simulink model "Mission_Server_Swarm_3QDrone_Vicon"  (Simulink 10.1)
settings: Solver=ode2  StartTime=0.0  StopTime=inf  FixedStep=0.001  RelTol=1e-3  EnableMultiTasking=on
undefined symbols (not defined in the file): datetime, Host, localhost, m, qc_get_step_size, saved_data
libraries: quarc_library x38, simulink x9
(part 1 of 2)
settings Model: Creator=Admin  LastModifiedBy=glai  SimulationMode=external  ExtModeTrigDuration=10000
settings SolverCC: PositivePriorityOrder=on
settings DataIOCC: SaveFormat=Dataset
settings OptimizationCC: LifeSpan=auto
settings DebuggingCC: UnderspecifiedInitializationDetection=Simplified  MergeDetectMultiDrivingBlocksExec=error
settings HardwareCC: ProdBitPerPointer=64  ProdBitPerSizeT=64  ProdBitPerPtrDiffT=64  ProdLargestAtomicFloat=Float  ProdIntDivRoundTo=Zero  ProdEndianess=LittleEndian  ProdWordSize=64  ProdHWDeviceType=Intel->x86-64 (Windows64)
settings ModelReferenceCC: PropagateSignalLabelsOutOfModel=on
settings RTWCC: Description=QUARC Win64 Target Using Toolchain  SystemTargetFile=quarc_win64.tlc  TemplateMakefile=quarc_default_tmf  Toolchain=QUARC win64 | nmake (64-bit Windows)  BuildConfiguration=Faster Runs
settings STFCustomTargetCC: ConcurrentExecutionCompliant=on  UseToolchainInfoCompliant=on  SystemTargetFile=quarc_win64.tlc
settings GRTTargetCC: ParMdlRefBuildCompliant=off  CompOptLevelCompliant=off  MatFileLogging=off  CPPClassGenCompliant=off  ExtMode=on  ExtModeMexFile=quarc_comm  ExtModeMexArgs='-w -d %d -uri %u -URI_Host_V1 tcpip://localhost:18001 -URI_Host_V2 tcpip://localhost:18002 -URI_Host_V3 tcpip://localhost:18003'

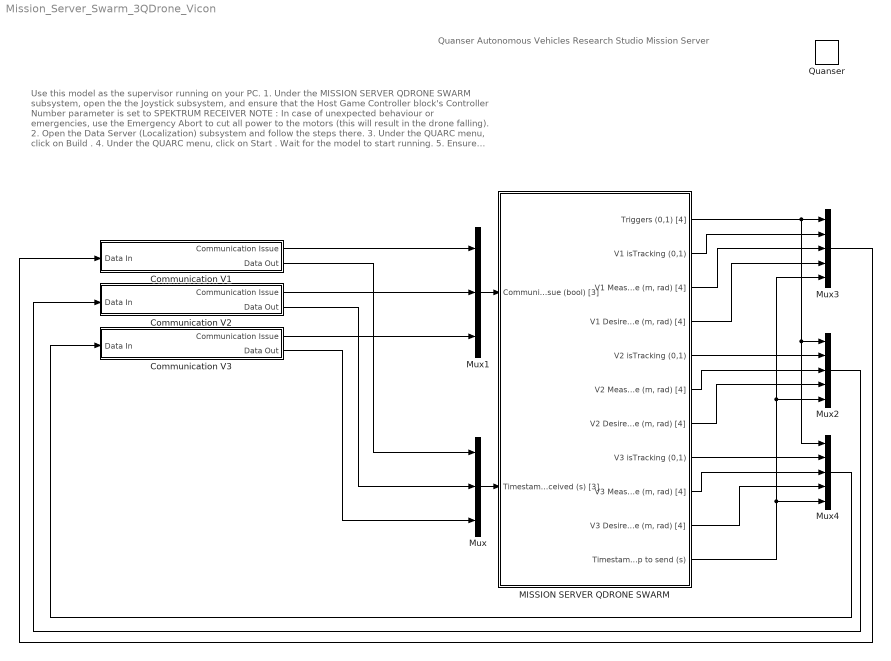
== system Mission_Server_Swarm_3QDrone_Vicon ==
  note: Use this model as the supervisor running on your PC.
      |
      | 1. Under the MISSION SERVER QDRONE SWARM subsystem, open the the Joystick subsystem, and ensure that the Host Game Controller block's Controller Number parameter is set to SPEKTRUM RECEIVER
      | NOTE : In case of unexpected behaviour or emergencies, use the Emergency Abort to cut all power to the motors (this will result in the drone falling).
      | 2. Open the Data Server (Localization) subsystem and follow the steps there.
      | 3. Under the QUARC menu, click on Build .
      | 4. Under the QUARC menu, click on Start . Wait for the model to start running.
      | 5. Ensure that the isTracking? display shows 1 and that the Joystick Issue display shows 0 (joystick must be powered ON with USB dongle attached to the PC).
      | NOTE : that the Comm Issue with Commander display SHOULD display 0 until the Commander_Stabilizer model is running. When it is running, this display should show 1.
  note: Quanser Autonomous Vehicles Research Studio
      | Mission Server
  Communication V1 : Subsystem
  Communication V2 : Subsystem
  Communication V3 : Subsystem
  MISSION SERVER QDRONE SWARM : Subsystem
  Mux : Mux  Inputs=3
  Mux1 : Mux  Inputs=3
  Mux2 : Mux  Inputs=5
  Mux3 : Mux  Inputs=5
  Mux4 : Mux  Inputs=5
  Quanser : quarc_library/Logos/Quanser
  wires:
  Communication V1/1(Communication Issue) -> Mux1/1
  Communication V2/1(Communication Issue) -> Mux1/2
  Communication V3/1(Communication Issue) -> Mux1/3
  Communication V3/2(Data Out) -> Mux/3
  Communication V2/2(Data Out) -> Mux/2
  Communication V1/2(Data Out) -> Mux/1
  MISSION SERVER QDRONE SWARM/11(Timestamp to send (s)) -> Mux3/5, Mux2/5, Mux4/5
  Mux3/1 -> Communication V1/1(Data In)
  Mux2/1 -> Communication V2/1(Data In)
  Mux4/1 -> Communication V3/1(Data In)
  Mux1/1 -> MISSION SERVER QDRONE SWARM/1(Communication  Issue (bool) [3])
  Mux/1 -> MISSION SERVER QDRONE SWARM/2(Timestamps received (s) [3])
  MISSION SERVER QDRONE SWARM/3("V1 Measured  Pose (m, rad) [4]") -> Mux3/3
  MISSION SERVER QDRONE SWARM/4("V1 Desired  Pose (m, rad) [4]") -> Mux3/4
  MISSION SERVER QDRONE SWARM/6("V2 Measured  Pose (m, rad) [4]") -> Mux2/3
  MISSION SERVER QDRONE SWARM/7("V2 Desired  Pose (m, rad) [4]") -> Mux2/4
  MISSION SERVER QDRONE SWARM/9("V3 Measured  Pose (m, rad) [4]") -> Mux4/3
  MISSION SERVER QDRONE SWARM/10("V3 Desired  Pose (m, rad) [4]") -> Mux4/4
  MISSION SERVER QDRONE SWARM/1(Triggers (0,1) [4]) -> Mux3/1, Mux4/1, Mux2/1
  MISSION SERVER QDRONE SWARM/2(V1 isTracking (0,1)) -> Mux3/2
  MISSION SERVER QDRONE SWARM/5(V2 isTracking (0,1)) -> Mux2/2
  MISSION SERVER QDRONE SWARM/8(V3 isTracking (0,1)) -> Mux4/2

== system Mission_Server_Swarm_3QDrone_Vicon/Communication V1 ==
  note: Argument (-URI_Host_V1) is set at the MEX-file arguments
      | found at Model Configuration Properties > Code Generation > Interface
      |
      | Format:
      | tcpip://localhost:18001
  Data In : Inport
  Constant : Constant
  Detect Communication loss : Subsystem
  Model Argument : quarc_library/Sources/Signals/Model Argument  argument_name=URI_Host_V1  has_value=on  data_type_mode=Specify via dialog  data_type=char  max_length=80  default_value=0  default_string=tcpip://localhost:18001  variable_size=off
      settings: AttributesFormatString=(-%<argument_name>)  SourceProductName=QUARC Targets
  Stream Server : quarc_library/Communications/Basic/Stream Server  uri_source=External input port  uri=tcpip://localhost:18877  apply_uri_to_all_configs=off  send_buffer_size=1460  receive_buffer_size=1460  byte_order=little endian (Intel - LSB first)  optimization=Minimum latency  send_options=Send most recent data  receive_options=Receive most recent data  default_value=zeros(1,1)  sample_time=qc_get_step_size  active=off  implementation=Use blocking I/O in a separate thread  send_fifo_size=1000  receive_fifo_size=1000  send_priority=0  receive_priority=0  send_dimensions=off  receive_dimensions=off  max_dimensions=-1  data_type=Inherited via back propagation  type_expr=BusObject
  "String Display " : quarc_library/Strings/String Display  alignment=center  display_mode=Single line  sample_time=-1  use_new=off
      settings: SourceProductName=QUARC Targets
  Terminator1 : Terminator
  Terminator2 : Terminator
  Communication Issue : Outport  VectorParamsAs1DForOutWhenUnconnected=off
  Data Out : Outport  Port=2  VectorParamsAs1DForOutWhenUnconnected=off
  wires:
  Detect Communication loss/1(Communication Issue (0,1)) -> Communication Issue/1
  Stream Server/1 -> Detect Communication loss/1(State)
  Stream Server/2 -> Detect Communication loss/2(Error)
  Stream Server/4 -> Data Out/1
  Model Argument/1 -> Stream Server/3, "String Display "/1
  Stream Server/5 -> Terminator1/1
  Stream Server/3 -> Terminator2/1
  Data In/1 -> Stream Server/1
  Constant/1 -> Stream Server/2

== system Mission_Server_Swarm_3QDrone_Vicon/Communication V2 ==
  note: Argument (-URI_Host_V2) is set at the MEX-file arguments
      | found at Model Configuration Properties > Code Generation > Interface
      |
      | Format:
      | tcpip://localhost:18002
  Data In : Inport
  Constant : Constant
  Detect Communication loss : Subsystem
  Model Argument : quarc_library/Sources/Signals/Model Argument  argument_name=URI_Host_V2  has_value=on  data_type_mode=Specify via dialog  data_type=char  max_length=80  default_value=0  default_string=tcpip://localhost:18002  variable_size=off
      settings: AttributesFormatString=(-%<argument_name>)  SourceProductName=QUARC Targets
  Stream Server : quarc_library/Communications/Basic/Stream Server  uri_source=External input port  uri=tcpip://localhost:18877  apply_uri_to_all_configs=off  send_buffer_size=1460  receive_buffer_size=1460  byte_order=little endian (Intel - LSB first)  optimization=Minimum latency  send_options=Send most recent data  receive_options=Receive most recent data  default_value=zeros(1,1)  sample_time=qc_get_step_size  active=off  implementation=Use blocking I/O in a separate thread  send_fifo_size=1000  receive_fifo_size=1000  send_priority=0  receive_priority=0  send_dimensions=off  receive_dimensions=off  max_dimensions=-1  data_type=Inherited via back propagation  type_expr=BusObject
  "String Display " : quarc_library/Strings/String Display  alignment=center  display_mode=Single line  sample_time=-1  use_new=off
      settings: SourceProductName=QUARC Targets
  Terminator1 : Terminator
  Terminator2 : Terminator
  Communication Issue : Outport  VectorParamsAs1DForOutWhenUnconnected=off
  Data Out : Outport  Port=2  VectorParamsAs1DForOutWhenUnconnected=off
  wires:
  Constant/1 -> Stream Server/2
  Data In/1 -> Stream Server/1
  Stream Server/3 -> Terminator2/1
  Stream Server/5 -> Terminator1/1
  Model Argument/1 -> "String Display "/1, Stream Server/3
  Stream Server/4 -> Data Out/1
  Stream Server/2 -> Detect Communication loss/2(Error)
  Stream Server/1 -> Detect Communication loss/1(State)
  Detect Communication loss/1(Communication Issue (0,1)) -> Communication Issue/1

== system Mission_Server_Swarm_3QDrone_Vicon/Communication V3 ==
  note: Argument (-URI_Host_V3) is set at the MEX-file arguments
      | found at Model Configuration Properties > Code Generation > Interface
      |
      | Format:
      | tcpip://localhost:18003
  Data In : Inport
  Constant : Constant
  Detect Communication loss : Subsystem
  Model Argument : quarc_library/Sources/Signals/Model Argument  argument_name=URI_Host_V3  has_value=on  data_type_mode=Specify via dialog  data_type=char  max_length=80  default_value=0  default_string=tcpip://localhost:18003  variable_size=off
      settings: AttributesFormatString=(-%<argument_name>)  SourceProductName=QUARC Targets
  Stream Server : quarc_library/Communications/Basic/Stream Server  uri_source=External input port  uri=tcpip://localhost:18877  apply_uri_to_all_configs=off  send_buffer_size=1460  receive_buffer_size=1460  byte_order=little endian (Intel - LSB first)  optimization=Minimum latency  send_options=Send most recent data  receive_options=Receive most recent data  default_value=zeros(1,1)  sample_time=qc_get_step_size  active=off  implementation=Use blocking I/O in a separate thread  send_fifo_size=1000  receive_fifo_size=1000  send_priority=0  receive_priority=0  send_dimensions=off  receive_dimensions=off  max_dimensions=-1  data_type=Inherited via back propagation  type_expr=BusObject
  "String Display " : quarc_library/Strings/String Display  alignment=center  display_mode=Single line  sample_time=-1  use_new=off
      settings: SourceProductName=QUARC Targets
  Terminator1 : Terminator
  Terminator2 : Terminator
  Communication Issue : Outport  VectorParamsAs1DForOutWhenUnconnected=off
  Data Out : Outport  Port=2  VectorParamsAs1DForOutWhenUnconnected=off
  wires:
  Detect Communication loss/1(Communication Issue (0,1)) -> Communication Issue/1
  Stream Server/1 -> Detect Communication loss/1(State)
  Stream Server/2 -> Detect Communication loss/2(Error)
  Stream Server/4 -> Data Out/1
  Model Argument/1 -> Stream Server/3, "String Display "/1
  Stream Server/5 -> Terminator1/1
  Stream Server/3 -> Terminator2/1
  Data In/1 -> Stream Server/1
  Constant/1 -> Stream Server/2

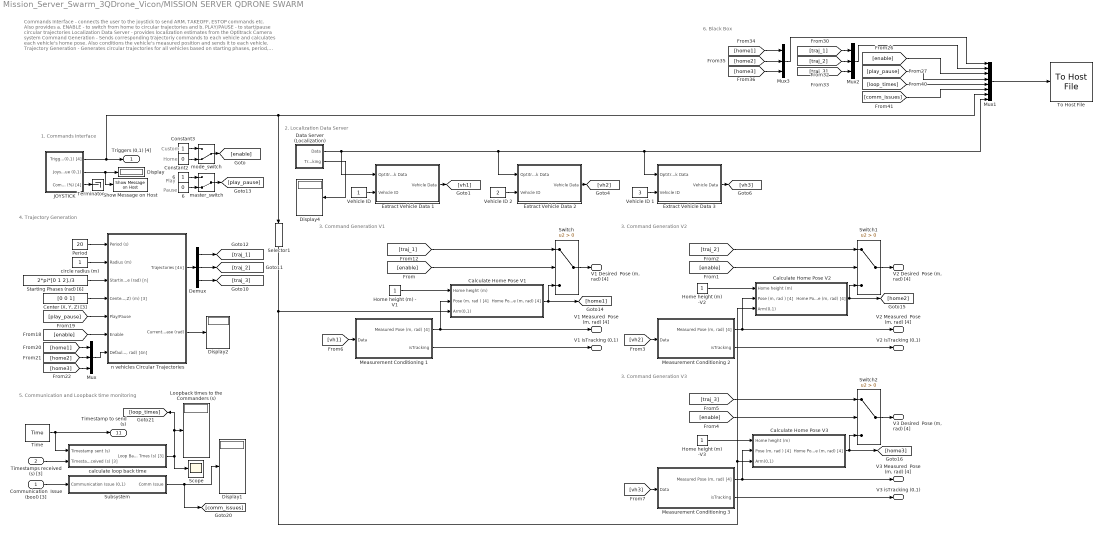
== system Mission_Server_Swarm_3QDrone_Vicon/MISSION SERVER QDRONE SWARM ==
  note: Commands Interface - connects the user to the joystick to send ARM, TAKEOFF, ESTOP commands etc. Also provides
      | a. ENABLE - to switch from home to circular trajectories and
      | b. PLAY/PAUSE - to start/pause circular trajectories
      | Localization Data Server - provides localization estimates from the Optitrack Camera system
      | Command Generation - Sends corresponding trajectoriy commands to each vehicle and calculates each vehicle's home pose. Also conditions the vehicle's measured position and sends it to each vehicle.
      | Trajectory Generation - Generates circular trajectories for all vehicles based on starting phases, period, radus and center location. When ENABLE is low, it switches to the trajectory at the Default (m, rad) [4] input
      | Communication and Loopback time monitoring - monitors communication issues with any vehicle, and also displays the loopback time to each model (time taken to send a packet to a vehicle and receive it back immediately).
      | Black Box: Logs selected data into log file for offline review and analysis.
  note: 6. Black Box
  note: 5. Communication and Loopback time monitoring
  note: 4. Trajectory Generation
  note: 2. Localization Data Server
  note: 1. Commands Interface
  note: Home
  note: Custom
  note: 3. Command Generation V1
  note: 3. Command Generation V2
  note: 3. Command Generation V3
  note: Pause
  note: Play
  Communication  Issue (bool) [3] : Inport
  Timestamps received (s) [3] : Inport  Port=2
  "          6" : Constant
  "   6" : Constant  Value=0
  Calculate Home Pose V1 : Subsystem
  Calculate Home Pose V2 : Subsystem
  Calculate Home Pose V3 : Subsystem
  "Center (X, Y, Z) [3]" : Constant  Value=[0 0 1]
  Constant2 : Constant  Value=0
  Constant3 : Constant
  "Data Server (Localization) " : Subsystem
  Demux : Demux  Outputs=[4 4 4 ]
  Display{,1..2,4} (4 alike) : Display
  Extract Vehicle Data 1 : Subsystem
  Extract Vehicle Data 2 : Subsystem
  Extract Vehicle Data 3 : Subsystem
  Home height (m) - V1 : Constant
  Home height (m) -V2 : Constant
  Home height (m) -V3 : Constant
  JOYSTICK : Subsystem
  Loopback times to the Commanders (s) : Display
  Measurement Conditioning 1 : Subsystem
  Measurement Conditioning 2 : Subsystem
  Measurement Conditioning 3 : Subsystem
  Mux : Mux  Inputs=3
  Mux1 : Mux  Inputs=8
  Mux2 : Mux  Inputs=3
  Mux3 : Mux  Inputs=3
  Period : Constant  Value=20
  Scope : Scope
  Selector1 : Selector  InputPortWidth=4  IndexOptions=Index vector (dialog)  Indices=[1]  OutputSizes=1
  "Show Message on Host " : quarc_library/Sinks/Error Handling/Show Message on Host  message_type=Fixed error message  message_icon=Warning  message=Mission Server: Joystick Disconnected
      settings: AttributesFormatString="\"%<message>\""  SourceProductName=QUARC Targets
  Starting Phases (rad) [6] : Constant  Value=2*pi*[0 1 2]./3
  Subsystem : Subsystem
  Switch : Switch  Criteria=u2 > Threshold
  Switch1 : Switch  Criteria=u2 > Threshold
  Switch2 : Switch  Criteria=u2 > Threshold
  Terminator : Terminator
  Time : quarc_library/Sources/Time/Time  time_source=Wall clock  sample_time=qc_get_step_size
  To Host File : quarc_library/Sinks/To Host/To Host File  file_name=saved_data/%m/%{char(datetime)}.mat  variable_name=data  decimation=1  sample_time=-1  file_format=MAT-file v.4  options=No header or footer  append=off  final_file_name=saved_data/Mission_Server_Swarm_3QDrone_Vicon/2022-03-11 10-34-30.mat  bitrate=2000000
  Vehicle ID : Constant
  Vehicle ID 1 : Constant  Value=3
  "Vehicle ID 2 " : Constant  Value=2
  calculate loop back time : Subsystem
  circle radius (m) : Constant
  master_switch : ManualSwitch  CurrentSetting=0
  mode_switch : ManualSwitch  CurrentSetting=0
  n vehicles Circular Trajectories : Subsystem
  Triggers (0,1) [4] : Outport  VectorParamsAs1DForOutWhenUnconnected=off
  V1 isTracking (0,1) : Outport  Port=2  VectorParamsAs1DForOutWhenUnconnected=off
  "V1 Measured  Pose (m, rad) [4]" : Outport  Port=3  VectorParamsAs1DForOutWhenUnconnected=off
  "V1 Desired  Pose (m, rad) [4]" : Outport  Port=4  VectorParamsAs1DForOutWhenUnconnected=off
  V2 isTracking (0,1) : Outport  Port=5  VectorParamsAs1DForOutWhenUnconnected=off
  "V2 Measured  Pose (m, rad) [4]" : Outport  Port=6  VectorParamsAs1DForOutWhenUnconnected=off
  "V2 Desired  Pose (m, rad) [4]" : Outport  Port=7  VectorParamsAs1DForOutWhenUnconnected=off
  V3 isTracking (0,1) : Outport  Port=8  VectorParamsAs1DForOutWhenUnconnected=off
  "V3 Measured  Pose (m, rad) [4]" : Outport  Port=9  VectorParamsAs1DForOutWhenUnconnected=off
  "V3 Desired  Pose (m, rad) [4]" : Outport  Port=10  VectorParamsAs1DForOutWhenUnconnected=off
  Timestamp to send (s) : Outport  Port=11  VectorParamsAs1DForOutWhenUnconnected=off
  wires:
  JOYSTICK/2(Joystick Issue (0,1)) -> Display/1, "Show Message on Host "/1
  Constant3/1 -> mode_switch/1
  Constant2/1 -> mode_switch/2
  JOYSTICK/3(Commands (%) [4]) -> Terminator/1
  "   6"/1 -> master_switch/2
  Period/1 -> n vehicles Circular Trajectories/1(Period (s))
  circle radius (m)/1 -> n vehicles Circular Trajectories/2(Radius (m))
  "          6"/1 -> master_switch/1
  [play_pause] -> n vehicles Circular Trajectories/5(Play/Pause)
  JOYSTICK/1(Triggers (0,1) [4]) -> Mux1/7, Selector1/1, Triggers (0,1) [4]/1
  "Data Server (Localization) "/2(Tracking) -> Display4/1
  Time/1 -> Timestamp to send (s)/1, calculate loop back time/1(Timestamp sent (s))
  Timestamps received (s) [3]/1 -> calculate loop back time/2(Timestamps received (s) [3])
  Starting Phases (rad) [6]/1 -> n vehicles Circular Trajectories/3(Starting Phase (rad) [n])
  "Center (X, Y, Z) [3]"/1 -> n vehicles Circular Trajectories/4(Center (X,Y,Z) (m) [3])
  n vehicles Circular Trajectories/2(Current Phase (rad)) -> Display2/1
  Vehicle ID 1/1 -> Extract Vehicle Data 3/2(Vehicle ID)
  "Vehicle ID 2 "/1 -> Extract Vehicle Data 2/2(Vehicle ID)
  Vehicle ID/1 -> Extract Vehicle Data 1/2(Vehicle ID)
  Measurement Conditioning 1/2(isTracking) -> V1 isTracking (0,1)/1
  Calculate Home Pose V1/1("Home Pose (m, rad) [4]") -> [home1], Switch/3
  [traj_1] -> Switch/1
  Home height (m) - V1/1 -> Calculate Home Pose V1/1(Home height (m))
  Measurement Conditioning 1/1("Measured Pose (m, rad) [4]") -> Calculate Home Pose V1/2("Pose (m, rad ) [4]"), "V1 Measured  Pose (m, rad) [4]"/1
  Switch/1 -> "V1 Desired  Pose (m, rad) [4]"/1
  mode_switch/1 -> [enable]
  [enable] -> Switch/2
  Extract Vehicle Data 1/1(Vehicle Data) -> [vh1]
  Extract Vehicle Data 2/1(Vehicle Data) -> [vh2]
  Extract Vehicle Data 3/1(Vehicle Data) -> [vh3]
  [vh1] -> Measurement Conditioning 1/1(Data)
  n vehicles Circular Trajectories/1(Trajectories [4n]) -> Demux/1
  Demux/1 -> [traj_1]
  Demux/2 -> [traj_2]
  Demux/3 -> [traj_3]
  [vh2] -> Measurement Conditioning 2/1(Data)
  [enable] -> Switch1/2
  Switch1/1 -> "V2 Desired  Pose (m, rad) [4]"/1
  Measurement Conditioning 2/1("Measured Pose (m, rad) [4]") -> Calculate Home Pose V2/2("Pose (m, rad ) [4]"), "V2 Measured  Pose (m, rad) [4]"/1
  Home height (m) -V2/1 -> Calculate Home Pose V2/1(Home height (m))
  [traj_2] -> Switch1/1
  Calculate Home Pose V2/1("Home Pose (m, rad) [4]") -> [home2], Switch1/3
  Measurement Conditioning 2/2(isTracking) -> V2 isTracking (0,1)/1
  Measurement Conditioning 3/2(isTracking) -> V3 isTracking (0,1)/1
  Calculate Home Pose V3/1("Home Pose (m, rad) [4]") -> [home3], Switch2/3
  [traj_3] -> Switch2/1
  Home height (m) -V3/1 -> Calculate Home Pose V3/1(Home height (m))
  Measurement Conditioning 3/1("Measured Pose (m, rad) [4]") -> Calculate Home Pose V3/2("Pose (m, rad ) [4]"), "V3 Measured  Pose (m, rad) [4]"/1
  Switch2/1 -> "V3 Desired  Pose (m, rad) [4]"/1
  [enable] -> Switch2/2
  [vh3] -> Measurement Conditioning 3/1(Data)
  [enable] -> n vehicles Circular Trajectories/6(Enable)
  master_switch/1 -> [play_pause]
  Communication  Issue (bool) [3]/1 -> Subsystem/1(Communication Issue (0,1))
  calculate loop back time/1(Loop Back Tmes (s) [3]) -> Scope/1, Loopback times to the Commanders (s)/1, [loop_times]
  Mux/1 -> n vehicles Circular Trajectories/7("Default (m, rad) [4n]")
  [home2] -> Mux/2
  [home3] -> Mux/3
  [home1] -> Mux/1
  Mux1/1 -> To Host File/1
  [play_pause] -> Mux1/4
  [enable] -> Mux1/3
  Mux2/1 -> Mux1/2
  [home1] -> Mux3/1
  [home3] -> Mux3/3
  [home2] -> Mux3/2
  [traj_3] -> Mux2/3
  [traj_2] -> Mux2/2
  [traj_1] -> Mux2/1
  Mux3/1 -> Mux1/1
  Subsystem/1(Comm Issue) -> [comm_issues], Display1/1
  [comm_issues] -> Mux1/6
  [loop_times] -> Mux1/5
  "Data Server (Localization) "/1(Data) -> Extract Vehicle Data 1/1(Optitrack Data), Extract Vehicle Data 2/1(Optitrack Data), Extract Vehicle Data 3/1(Optitrack Data), Mux1/8
  Selector1/1 -> Calculate Home Pose V3/3(Arm(0,1)), Calculate Home Pose V2/3(Arm(0,1)), Calculate Home Pose V1/3(Arm(0,1))

== system Mission_Server_Swarm_3QDrone_Vicon/Communication V1/Detect Communication loss ==
  State : Inport
  Error : Inport  Port=2
  Data Type Conversion : DataTypeConversion
  MATLAB Function : MATLAB Function  TreatAsAtomicUnit=on
  Terminator2 : Terminator
  Threshold : quarc_library/Discontinuities/Threshold  operator=>=  param_src=Specify via dialog  threshold=0.5  duration=0.1
      settings: SourceProductName=QUARC Targets
  Time : quarc_library/Sources/Time/Time  time_source=Wall clock  sample_time=qc_get_step_size
  Communication Issue (0,1) : Outport  VectorParamsAs1DForOutWhenUnconnected=off
  wires:
  Threshold/1 -> Data Type Conversion/1
  Data Type Conversion/1 -> Communication Issue (0,1)/1
  Threshold/2 -> Terminator2/1
  Time/1 -> MATLAB Function/1(time)
  State/1 -> MATLAB Function/2(state)
  MATLAB Function/1(stream_connection_loss) -> Threshold/1
  Error/1 -> MATLAB Function/3(error)

== system Mission_Server_Swarm_3QDrone_Vicon/Communication V2/Detect Communication loss ==
  State : Inport
  Error : Inport  Port=2
  Data Type Conversion : DataTypeConversion
  MATLAB Function : MATLAB Function  TreatAsAtomicUnit=on
  Terminator2 : Terminator
  Threshold : quarc_library/Discontinuities/Threshold  operator=>=  param_src=Specify via dialog  threshold=0.5  duration=0.1
      settings: SourceProductName=QUARC Targets
  Time : quarc_library/Sources/Time/Time  time_source=Wall clock  sample_time=qc_get_step_size
  Communication Issue (0,1) : Outport  VectorParamsAs1DForOutWhenUnconnected=off
  wires:
  Error/1 -> MATLAB Function/3(error)
  MATLAB Function/1(stream_connection_loss) -> Threshold/1
  State/1 -> MATLAB Function/2(state)
  Time/1 -> MATLAB Function/1(time)
  Threshold/2 -> Terminator2/1
  Data Type Conversion/1 -> Communication Issue (0,1)/1
  Threshold/1 -> Data Type Conversion/1

== system Mission_Server_Swarm_3QDrone_Vicon/Communication V3/Detect Communication loss ==
  State : Inport
  Error : Inport  Port=2
  Data Type Conversion : DataTypeConversion
  MATLAB Function : MATLAB Function  TreatAsAtomicUnit=on
  Terminator2 : Terminator
  Threshold : quarc_library/Discontinuities/Threshold  operator=>=  param_src=Specify via dialog  threshold=0.5  duration=0.1
      settings: SourceProductName=QUARC Targets
  Time : quarc_library/Sources/Time/Time  time_source=Wall clock  sample_time=qc_get_step_size
  Communication Issue (0,1) : Outport  VectorParamsAs1DForOutWhenUnconnected=off
  wires:
  Threshold/1 -> Data Type Conversion/1
  Data Type Conversion/1 -> Communication Issue (0,1)/1
  Threshold/2 -> Terminator2/1
  Time/1 -> MATLAB Function/1(time)
  State/1 -> MATLAB Function/2(state)
  MATLAB Function/1(stream_connection_loss) -> Threshold/1
  Error/1 -> MATLAB Function/3(error)

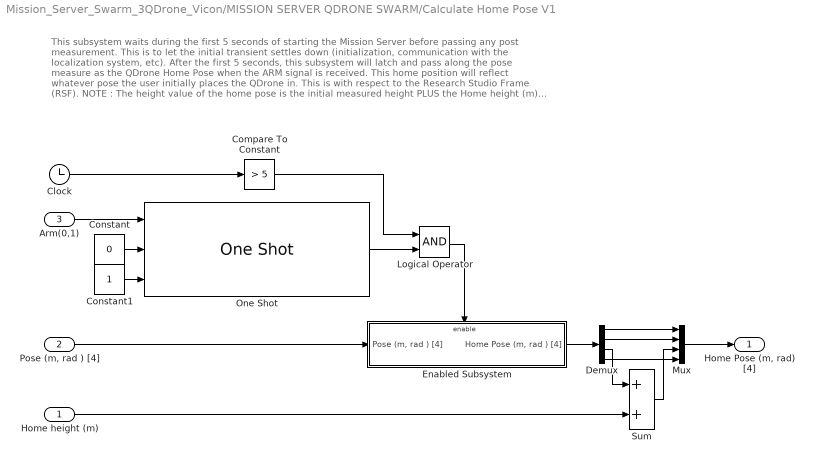
== system Mission_Server_Swarm_3QDrone_Vicon/MISSION SERVER QDRONE SWARM/Calculate Home Pose V1 ==
  note: This subsystem waits during the first 5 seconds of starting the Mission Server before passing any post measurement.
      | This is to let the initial transient settles down (initialization, communication with the localization system, etc).
      | After the first 5 seconds, this subsystem will latch and pass along the pose measure as the QDrone Home Pose when
      | the ARM signal is received.
      | This home position will reflect whatever pose the user initially places the QDrone in.
      | This is with respect to the Research Studio Frame (RSF).
      |
      | NOTE : The height value of the home pose is the initial measured height PLUS the Home height (m) input value.
  Home height (m) : Inport
  "Pose (m, rad ) [4]" : Inport  Port=2
  Arm(0,1) : Inport  Port=3
  Clock : Clock
  Compare To Constant : simulink/Logic and Bit Operations/Compare To Constant  relop=>  const=5  OutDataTypeStr=boolean
  Constant : Constant  Value=0
  Constant1 : Constant
  Demux : Demux
  Enabled Subsystem : Subsystem  TreatAsAtomicUnit=on
  Logical Operator : Logic  AllPortsSameDT=off  OutDataTypeStr=boolean
  Mux : Mux
  One Shot : quarc_library/Discontinuities/One Shot  trigger_type=Rising edge  redun_pulse=Ignore extraneous pulse  width_source=Specify via dialog  pulse_width=1/qc_get_step_size
      settings: SourceProductName=QUARC Targets
  Sum : Sum
  "Home Pose (m, rad) [4]" : Outport  VectorParamsAs1DForOutWhenUnconnected=off
  wires:
  Constant/1 -> One Shot/2
  Constant1/1 -> One Shot/3
  Arm(0,1)/1 -> One Shot/1
  One Shot/1 -> Logical Operator/2
  "Pose (m, rad ) [4]"/1 -> Enabled Subsystem/1("Pose (m, rad ) [4] ")
  Clock/1 -> Compare To Constant/1
  Compare To Constant/1 -> Logical Operator/1
  Logical Operator/1 -> Enabled Subsystem/Enable
  Enabled Subsystem/1("Home Pose (m, rad ) [4]") -> Demux/1
  Demux/1 -> Mux/1
  Demux/2 -> Mux/2
  Demux/4 -> Mux/4
  Demux/3 -> Sum/1
  Sum/1 -> Mux/3
  Home height (m)/1 -> Sum/2
  Mux/1 -> "Home Pose (m, rad) [4]"/1

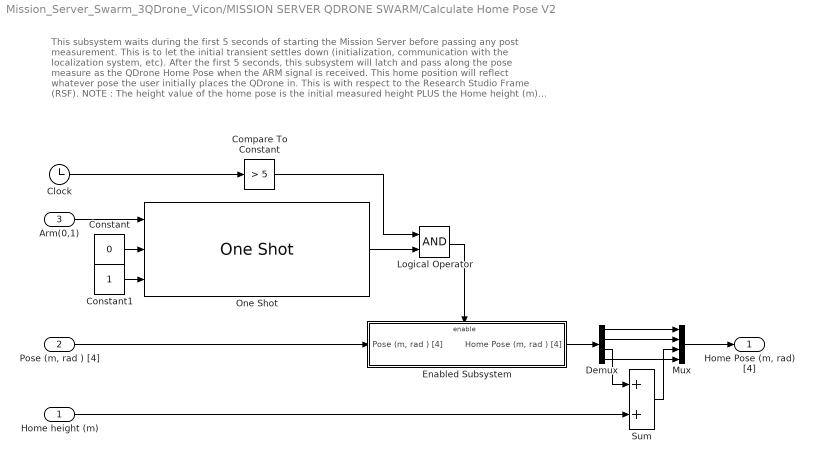
== system Mission_Server_Swarm_3QDrone_Vicon/MISSION SERVER QDRONE SWARM/Calculate Home Pose V2 ==
  note: This subsystem waits during the first 5 seconds of starting the Mission Server before passing any post measurement.
      | This is to let the initial transient settles down (initialization, communication with the localization system, etc).
      | After the first 5 seconds, this subsystem will latch and pass along the pose measure as the QDrone Home Pose when
      | the ARM signal is received.
      | This home position will reflect whatever pose the user initially places the QDrone in.
      | This is with respect to the Research Studio Frame (RSF).
      |
      | NOTE : The height value of the home pose is the initial measured height PLUS the Home height (m) input value.
  Home height (m) : Inport
  "Pose (m, rad ) [4]" : Inport  Port=2
  Arm(0,1) : Inport  Port=3
  Clock : Clock
  Compare To Constant : simulink/Logic and Bit Operations/Compare To Constant  relop=>  const=5  OutDataTypeStr=boolean
  Constant : Constant  Value=0
  Constant1 : Constant
  Demux : Demux
  Enabled Subsystem : Subsystem  TreatAsAtomicUnit=on
  Logical Operator : Logic  AllPortsSameDT=off  OutDataTypeStr=boolean
  Mux : Mux
  One Shot : quarc_library/Discontinuities/One Shot  trigger_type=Rising edge  redun_pulse=Ignore extraneous pulse  width_source=Specify via dialog  pulse_width=1/qc_get_step_size
      settings: SourceProductName=QUARC Targets
  Sum : Sum
  "Home Pose (m, rad) [4]" : Outport  VectorParamsAs1DForOutWhenUnconnected=off
  wires:
  Mux/1 -> "Home Pose (m, rad) [4]"/1
  Home height (m)/1 -> Sum/2
  Sum/1 -> Mux/3
  Demux/3 -> Sum/1
  Demux/4 -> Mux/4
  Demux/2 -> Mux/2
  Demux/1 -> Mux/1
  Enabled Subsystem/1("Home Pose (m, rad ) [4]") -> Demux/1
  Logical Operator/1 -> Enabled Subsystem/Enable
  Compare To Constant/1 -> Logical Operator/1
  Clock/1 -> Compare To Constant/1
  "Pose (m, rad ) [4]"/1 -> Enabled Subsystem/1("Pose (m, rad ) [4] ")
  One Shot/1 -> Logical Operator/2
  Arm(0,1)/1 -> One Shot/1
  Constant1/1 -> One Shot/3
  Constant/1 -> One Shot/2

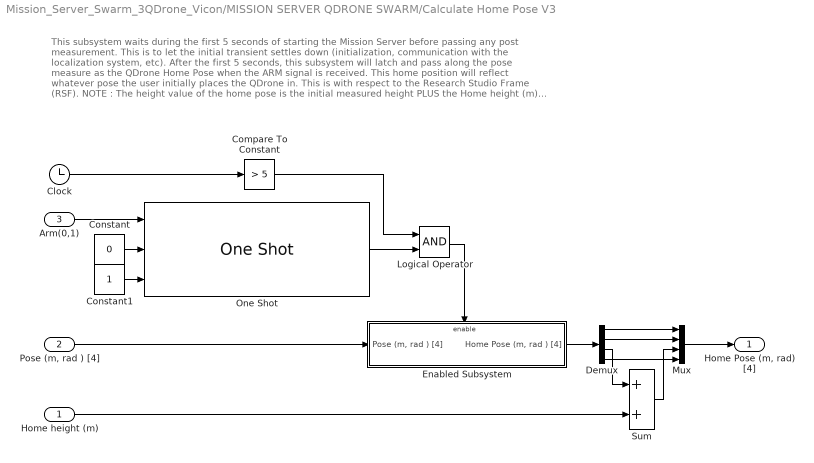
== system Mission_Server_Swarm_3QDrone_Vicon/MISSION SERVER QDRONE SWARM/Calculate Home Pose V3 ==
  note: This subsystem waits during the first 5 seconds of starting the Mission Server before passing any post measurement.
      | This is to let the initial transient settles down (initialization, communication with the localization system, etc).
      | After the first 5 seconds, this subsystem will latch and pass along the pose measure as the QDrone Home Pose when
      | the ARM signal is received.
      | This home position will reflect whatever pose the user initially places the QDrone in.
      | This is with respect to the Research Studio Frame (RSF).
      |
      | NOTE : The height value of the home pose is the initial measured height PLUS the Home height (m) input value.
  Home height (m) : Inport
  "Pose (m, rad ) [4]" : Inport  Port=2
  Arm(0,1) : Inport  Port=3
  Clock : Clock
  Compare To Constant : simulink/Logic and Bit Operations/Compare To Constant  relop=>  const=5  OutDataTypeStr=boolean
  Constant : Constant  Value=0
  Constant1 : Constant
  Demux : Demux
  Enabled Subsystem : Subsystem  TreatAsAtomicUnit=on
  Logical Operator : Logic  AllPortsSameDT=off  OutDataTypeStr=boolean
  Mux : Mux
  One Shot : quarc_library/Discontinuities/One Shot  trigger_type=Rising edge  redun_pulse=Ignore extraneous pulse  width_source=Specify via dialog  pulse_width=1/qc_get_step_size
      settings: SourceProductName=QUARC Targets
  Sum : Sum
  "Home Pose (m, rad) [4]" : Outport  VectorParamsAs1DForOutWhenUnconnected=off
  wires:
  Mux/1 -> "Home Pose (m, rad) [4]"/1
  Home height (m)/1 -> Sum/2
  Sum/1 -> Mux/3
  Demux/3 -> Sum/1
  Demux/4 -> Mux/4
  Demux/2 -> Mux/2
  Demux/1 -> Mux/1
  Enabled Subsystem/1("Home Pose (m, rad ) [4]") -> Demux/1
  Logical Operator/1 -> Enabled Subsystem/Enable
  Compare To Constant/1 -> Logical Operator/1
  Clock/1 -> Compare To Constant/1
  "Pose (m, rad ) [4]"/1 -> Enabled Subsystem/1("Pose (m, rad ) [4] ")
  One Shot/1 -> Logical Operator/2
  Arm(0,1)/1 -> One Shot/1
  Constant1/1 -> One Shot/3
  Constant/1 -> One Shot/2

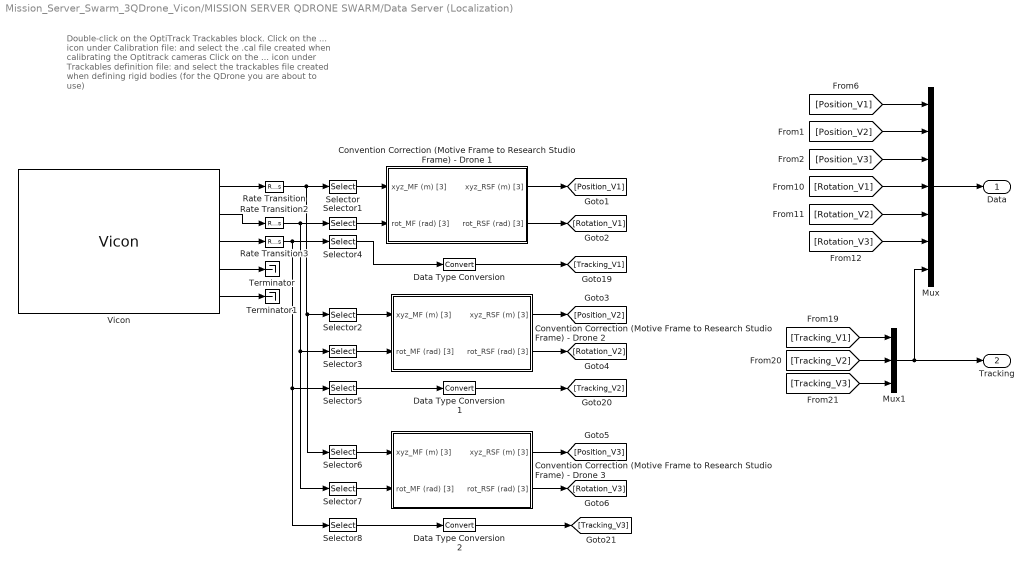
== system Mission_Server_Swarm_3QDrone_Vicon/MISSION SERVER QDRONE SWARM/Data Server (Localization)  ==
  note: Double-click on the OptiTrack Trackables block.
      |
      | Click on the ... icon under Calibration file: and select the .cal file
      | created when calibrating the Optitrack cameras
      |
      | Click on the ... icon under Trackables definition file: and select
      | the trackables file created when defining rigid bodies (for the
      | QDrone you are about to use)
  Convention Correction (Motive Frame to Research Studio Frame) - Drone 1 : Subsystem
  Convention Correction (Motive Frame to Research Studio Frame) - Drone 2 : Subsystem
  Convention Correction (Motive Frame to Research Studio Frame) - Drone 3 : Subsystem
  Data Type Conversion : DataTypeConversion
  Data Type Conversion1 : DataTypeConversion
  Data Type Conversion2 : DataTypeConversion
  Mux : Mux  Inputs=7
  Mux1 : Mux  Inputs=3
  Rate Transition : RateTransition
  Rate Transition2 : RateTransition
  Rate Transition3 : RateTransition
  Selector : Selector  InputPortWidth=9  IndexOptions=Index vector (dialog)  Indices=[1:3]  OutputSizes=1
  Selector1 : Selector  InputPortWidth=9  IndexOptions=Index vector (dialog)  Indices=[1:3]  OutputSizes=1
  Selector2 : Selector  InputPortWidth=9  IndexOptions=Index vector (dialog)  Indices=[4:6]  OutputSizes=1
  Selector3 : Selector  InputPortWidth=9  IndexOptions=Index vector (dialog)  Indices=[4:6]  OutputSizes=1
  Selector4 : Selector  InputPortWidth=3  IndexOptions=Index vector (dialog)  Indices=[1]  OutputSizes=1
  Selector5 : Selector  InputPortWidth=3  IndexOptions=Index vector (dialog)  Indices=[2]  OutputSizes=1
  Selector6 : Selector  InputPortWidth=9  IndexOptions=Index vector (dialog)  Indices=[7:9]  OutputSizes=1
  Selector7 : Selector  InputPortWidth=9  IndexOptions=Index vector (dialog)  Indices=[7:9]  OutputSizes=1
  Selector8 : Selector  InputPortWidth=3  IndexOptions=Index vector (dialog)  Indices=[3]  OutputSizes=1
  Terminator : Terminator
  Terminator1 : Terminator
  Vicon : quarc_library/Devices/Third-Party/Vicon/Vicon  hostname=localhost:801  segment_list=ObjectName.ObjectName\0ObjectName.ObjectName\0ObjectName.ObjectName\0\0  marker_list=\0  unlabeled_markers=[]  stream_mode=2  sample_time=qc_get_step_size  num_segments=3  num_markers=0  active=on
      settings: SourceProductName=QUARC Targets
  Data : Outport  VectorParamsAs1DForOutWhenUnconnected=off
  Tracking : Outport  Port=2  VectorParamsAs1DForOutWhenUnconnected=off
  wires:
  Vicon/3 -> Rate Transition3/1
  Mux/1 -> Data/1
  Vicon/1 -> Rate Transition/1
  Vicon/2 -> Rate Transition2/1
  Selector/1 -> Convention Correction (Motive Frame to Research Studio Frame) - Drone 1/1(xyz_MF (m) [3])
  Selector1/1 -> Convention Correction (Motive Frame to Research Studio Frame) - Drone 1/2(rot_MF (rad) [3])
  Selector2/1 -> Convention Correction (Motive Frame to Research Studio Frame) - Drone 2/1(xyz_MF (m) [3])
  Selector3/1 -> Convention Correction (Motive Frame to Research Studio Frame) - Drone 2/2(rot_MF (rad) [3])
  Selector4/1 -> Data Type Conversion/1
  Selector5/1 -> Data Type Conversion1/1
  Selector8/1 -> Data Type Conversion2/1
  Selector7/1 -> Convention Correction (Motive Frame to Research Studio Frame) - Drone 3/2(rot_MF (rad) [3])
  Selector6/1 -> Convention Correction (Motive Frame to Research Studio Frame) - Drone 3/1(xyz_MF (m) [3])
  Rate Transition2/1 -> Selector1/1, Selector7/1, Selector3/1
  Rate Transition3/1 -> Selector4/1, Selector8/1, Selector5/1
  Rate Transition/1 -> Selector6/1, Selector2/1, Selector/1
  Convention Correction (Motive Frame to Research Studio Frame) - Drone 1/1(xyz_RSF (m) [3]) -> [Position_V1]
  [Position_V1] -> Mux/1
  [Position_V2] -> Mux/2
  [Position_V3] -> Mux/3
  Convention Correction (Motive Frame to Research Studio Frame) - Drone 1/2(rot_RSF (rad) [3]) -> [Rotation_V1]
  [Rotation_V3] -> Mux/6
  [Tracking_V1] -> Mux1/1
  [Tracking_V2] -> Mux1/2
  [Tracking_V3] -> Mux1/3
  Convention Correction (Motive Frame to Research Studio Frame) - Drone 2/1(xyz_RSF (m) [3]) -> [Position_V2]
  Convention Correction (Motive Frame to Research Studio Frame) - Drone 2/2(rot_RSF (rad) [3]) -> [Rotation_V2]
  Convention Correction (Motive Frame to Research Studio Frame) - Drone 3/1(xyz_RSF (m) [3]) -> [Position_V3]
  Convention Correction (Motive Frame to Research Studio Frame) - Drone 3/2(rot_RSF (rad) [3]) -> [Rotation_V3]
  Data Type Conversion/1 -> [Tracking_V1]
  Data Type Conversion1/1 -> [Tracking_V2]
  Data Type Conversion2/1 -> [Tracking_V3]
  Mux1/1 -> Tracking/1, Mux/7
  [Rotation_V1] -> Mux/4
  [Rotation_V2] -> Mux/5
  Vicon/4 -> Terminator/1
  Vicon/5 -> Terminator1/1

== system Mission_Server_Swarm_3QDrone_Vicon/MISSION SERVER QDRONE SWARM/Extract Vehicle Data 1 ==
  Optitrack Data : Inport
  Vehicle ID : Inport  Port=2
  Data Type Conversion10 : DataTypeConversion
  Data Type Conversion11 : DataTypeConversion
  Data Type Conversion9 : DataTypeConversion
  Extract Object Data : MATLAB Function  TreatAsAtomicUnit=on
  Mux1 : Mux  Inputs=3
  Reshape : Reshape
  Reshape1 : Reshape
  Reshape2 : Reshape
  Vehicle Data : Outport  VectorParamsAs1DForOutWhenUnconnected=off
  wires:
  Reshape2/1 -> Data Type Conversion9/1
  Reshape1/1 -> Data Type Conversion10/1
  Reshape/1 -> Data Type Conversion11/1
  Data Type Conversion9/1 -> Mux1/3
  Data Type Conversion10/1 -> Mux1/2
  Data Type Conversion11/1 -> Mux1/1
  Extract Object Data/2(orientation) -> Reshape1/1
  Extract Object Data/3(tracking) -> Reshape2/1
  Extract Object Data/1(position) -> Reshape/1
  Mux1/1 -> Vehicle Data/1
  Optitrack Data/1 -> Extract Object Data/1(data)
  Vehicle ID/1 -> Extract Object Data/2(index)

== system Mission_Server_Swarm_3QDrone_Vicon/MISSION SERVER QDRONE SWARM/Extract Vehicle Data 2 ==
  Optitrack Data : Inport
  Vehicle ID : Inport  Port=2
  Data Type Conversion10 : DataTypeConversion
  Data Type Conversion11 : DataTypeConversion
  Data Type Conversion9 : DataTypeConversion
  Display : Display
  Display1 : Display
  Extract Object Data : MATLAB Function  TreatAsAtomicUnit=on
  Mux1 : Mux  Inputs=3
  Reshape : Reshape
  Reshape1 : Reshape
  Reshape2 : Reshape
  Vehicle Data : Outport  VectorParamsAs1DForOutWhenUnconnected=off
  wires:
  Vehicle ID/1 -> Extract Object Data/2(index)
  Optitrack Data/1 -> Extract Object Data/1(data)
  Mux1/1 -> Vehicle Data/1
  Extract Object Data/1(position) -> Display/1, Reshape/1
  Extract Object Data/3(tracking) -> Reshape2/1
  Extract Object Data/2(orientation) -> Display1/1, Reshape1/1
  Data Type Conversion11/1 -> Mux1/1
  Data Type Conversion10/1 -> Mux1/2
  Data Type Conversion9/1 -> Mux1/3
  Reshape/1 -> Data Type Conversion11/1
  Reshape1/1 -> Data Type Conversion10/1
  Reshape2/1 -> Data Type Conversion9/1

== system Mission_Server_Swarm_3QDrone_Vicon/MISSION SERVER QDRONE SWARM/Extract Vehicle Data 3 ==
  Optitrack Data : Inport
  Vehicle ID : Inport  Port=2
  Data Type Conversion10 : DataTypeConversion
  Data Type Conversion11 : DataTypeConversion
  Data Type Conversion9 : DataTypeConversion
  Extract Object Data : MATLAB Function  TreatAsAtomicUnit=on
  Mux1 : Mux  Inputs=3
  Reshape : Reshape
  Reshape1 : Reshape
  Reshape2 : Reshape
  Vehicle Data : Outport  VectorParamsAs1DForOutWhenUnconnected=off
  wires:
  Vehicle ID/1 -> Extract Object Data/2(index)
  Optitrack Data/1 -> Extract Object Data/1(data)
  Mux1/1 -> Vehicle Data/1
  Extract Object Data/1(position) -> Reshape/1
  Extract Object Data/3(tracking) -> Reshape2/1
  Extract Object Data/2(orientation) -> Reshape1/1
  Data Type Conversion11/1 -> Mux1/1
  Data Type Conversion10/1 -> Mux1/2
  Data Type Conversion9/1 -> Mux1/3
  Reshape/1 -> Data Type Conversion11/1
  Reshape1/1 -> Data Type Conversion10/1
  Reshape2/1 -> Data Type Conversion9/1

== system Mission_Server_Swarm_3QDrone_Vicon/MISSION SERVER QDRONE SWARM/JOYSTICK ==
  note: Throttle
      | Roll
      | Pitch
      | Yaw
  Host Game Controller : quarc_library/Devices/Peripherals/Host/Host Game Controller  object_name=Host-1  controller=1  buffer_size=20  deadzone=[]  saturation=[]  sample_time=qc_get_step_size  auto_center=off  enabled=on  debug_mode=off
      settings: SourceProductName=QUARC Targets
  Host Initialize : quarc_library/Devices/Peripherals/Host/Host Initialize  object_name=Host-1  uri_source=Use external mode communications  uri=tcpip://localhost:18001  apply_uri_to_all_configs=on  send_buffer_size=1000  receive_buffer_size=1000  thread_priority=0  run_client=on  use_window=off  window_position=[]  sample_time=qc_get_step_size  active=on
      settings: SourceProductName=QUARC Targets
  Initialization and Conditioning : Subsystem  TreatAsAtomicUnit=on
  Pulse Check : Subsystem  TreatAsAtomicUnit=on
  Spectrum DXe Mapping : Subsystem
  Terminator{1..4} (4 alike) : Terminator
  Triggers (0,1) [4] : Outport  VectorParamsAs1DForOutWhenUnconnected=off
  Joystick Issue (0,1) : Outport  Port=2  VectorParamsAs1DForOutWhenUnconnected=off
  Commands (%) [4] : Outport  Port=3  VectorParamsAs1DForOutWhenUnconnected=off
  wires:
  Initialization and Conditioning/1(Joystick Issue (0,1)) -> Joystick Issue (0,1)/1
  Spectrum DXe Mapping/1(Joystick Issue (bool)) -> Initialization and Conditioning/1(Joystick Issue (bool))
  Host Game Controller/7 -> Spectrum DXe Mapping/7(Rx)
  Host Game Controller/10 -> Terminator3/1
  Host Game Controller/9 -> Terminator2/1
  Host Game Controller/8 -> Spectrum DXe Mapping/8(Ry)
  Host Game Controller/4 -> Spectrum DXe Mapping/4(x)
  Host Game Controller/5 -> Spectrum DXe Mapping/5(y)
  Host Game Controller/3 -> Spectrum DXe Mapping/3(Sliders)
  Host Game Controller/6 -> Spectrum DXe Mapping/6(z)
  Host Initialize/1 -> Terminator4/1
  Host Initialize/2 -> Terminator1/1
  Spectrum DXe Mapping/3(Yaw (%)) -> Initialization and Conditioning/3(Yaw (%))
  Spectrum DXe Mapping/7("Arm/Disarm (bool) ") -> Initialization and Conditioning/7(Arm/Disarm (bool))
  Spectrum DXe Mapping/5(Roll (%)) -> Initialization and Conditioning/5(Roll (%))
  Spectrum DXe Mapping/4(Throttle (%)) -> Initialization and Conditioning/4(Throttle (%))
  Spectrum DXe Mapping/6(Pitch (%)) -> Initialization and Conditioning/6(Pitch (%))
  Host Game Controller/2 -> Spectrum DXe Mapping/2(buttons)
  Spectrum DXe Mapping/2(Emergency Abort (bool)) -> Initialization and Conditioning/2(Emergency Abort (bool))
  Initialization and Conditioning/2(Triggers (0,1) [4]) -> Triggers (0,1) [4]/1
  Spectrum DXe Mapping/8(Takeoff/Autoland (bool)) -> Initialization and Conditioning/8(Takeoff/AutoLand (bool))
  Initialization and Conditioning/3(Commands (%) [4]) -> Commands (%) [4]/1
  Host Game Controller/1 -> Spectrum DXe Mapping/1(new), Pulse Check/1(new)
  Pulse Check/1(signal enable) -> Initialization and Conditioning/Enable

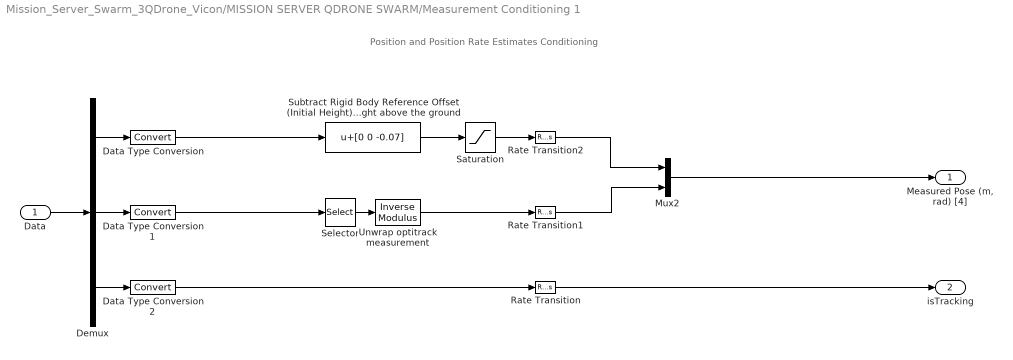
== system Mission_Server_Swarm_3QDrone_Vicon/MISSION SERVER QDRONE SWARM/Measurement Conditioning 1 ==
  note: Position and Position Rate Estimates Conditioning
  Data : Inport
  Data Type Conversion : DataTypeConversion
  Data Type Conversion1 : DataTypeConversion
  Data Type Conversion2 : DataTypeConversion
  Demux : Demux  Outputs=[3 3 1]
  Mux2 : Mux  Inputs=[3 1]
  Rate Transition : RateTransition
  Rate Transition1 : RateTransition
  Rate Transition2 : RateTransition
  Saturation : Saturate  UpperLimit=[2 2 5]  LowerLimit=[-2 -2 0]
  Selector : Selector  InputPortWidth=3  IndexOptions=Index vector (dialog)  Indices=[3]  OutputSizes=1
  Subtract Rigid Body Reference Offset (Initial Height)  to get height above the ground : Bias  Bias=[0 0 -0.07]
  Unwrap optitrack measurement : quarc_library/Discontinuities/Inverse Modulus  modulus=2*pi  output_derivative=off  output_revolutions=off  max_x=Inf  min_x=-Inf
  "Measured Pose (m, rad) [4]" : Outport  VectorParamsAs1DForOutWhenUnconnected=off
  isTracking : Outport  Port=2  VectorParamsAs1DForOutWhenUnconnected=off
  wires:
  Demux/2 -> Data Type Conversion1/1
  Demux/1 -> Data Type Conversion/1
  Demux/3 -> Data Type Conversion2/1
  Mux2/1 -> "Measured Pose (m, rad) [4]"/1
  Data Type Conversion2/1 -> Rate Transition/1
  Data/1 -> Demux/1
  Rate Transition/1 -> isTracking/1
  Subtract Rigid Body Reference Offset (Initial Height)  to get height above the ground/1 -> Saturation/1
  Rate Transition2/1 -> Mux2/1
  Saturation/1 -> Rate Transition2/1
  Data Type Conversion1/1 -> Selector/1
  Selector/1 -> Unwrap optitrack measurement/1
  Data Type Conversion/1 -> Subtract Rigid Body Reference Offset (Initial Height)  to get height above the ground/1
  Unwrap optitrack measurement/1 -> Rate Transition1/1
  Rate Transition1/1 -> Mux2/2

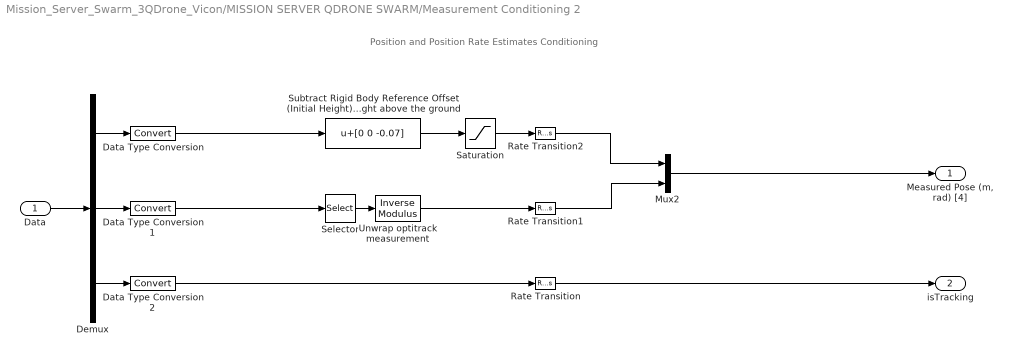
== system Mission_Server_Swarm_3QDrone_Vicon/MISSION SERVER QDRONE SWARM/Measurement Conditioning 2 ==
  note: Position and Position Rate Estimates Conditioning
  Data : Inport
  Data Type Conversion : DataTypeConversion
  Data Type Conversion1 : DataTypeConversion
  Data Type Conversion2 : DataTypeConversion
  Demux : Demux  Outputs=[3 3 1]
  Mux2 : Mux  Inputs=[3 1]
  Rate Transition : RateTransition
  Rate Transition1 : RateTransition
  Rate Transition2 : RateTransition
  Saturation : Saturate  UpperLimit=[2 2 5]  LowerLimit=[-2 -2 0]
  Selector : Selector  InputPortWidth=3  IndexOptions=Index vector (dialog)  Indices=[3]  OutputSizes=1
  Subtract Rigid Body Reference Offset (Initial Height)  to get height above the ground : Bias  Bias=[0 0 -0.07]
  Unwrap optitrack measurement : quarc_library/Discontinuities/Inverse Modulus  modulus=2*pi  output_derivative=off  output_revolutions=off  max_x=Inf  min_x=-Inf
  "Measured Pose (m, rad) [4]" : Outport  VectorParamsAs1DForOutWhenUnconnected=off
  isTracking : Outport  Port=2  VectorParamsAs1DForOutWhenUnconnected=off
  wires:
  Rate Transition1/1 -> Mux2/2
  Unwrap optitrack measurement/1 -> Rate Transition1/1
  Data Type Conversion/1 -> Subtract Rigid Body Reference Offset (Initial Height)  to get height above the ground/1
  Selector/1 -> Unwrap optitrack measurement/1
  Data Type Conversion1/1 -> Selector/1
  Saturation/1 -> Rate Transition2/1
  Rate Transition2/1 -> Mux2/1
  Subtract Rigid Body Reference Offset (Initial Height)  to get height above the ground/1 -> Saturation/1
  Rate Transition/1 -> isTracking/1
  Data/1 -> Demux/1
  Data Type Conversion2/1 -> Rate Transition/1
  Mux2/1 -> "Measured Pose (m, rad) [4]"/1
  Demux/3 -> Data Type Conversion2/1
  Demux/1 -> Data Type Conversion/1
  Demux/2 -> Data Type Conversion1/1

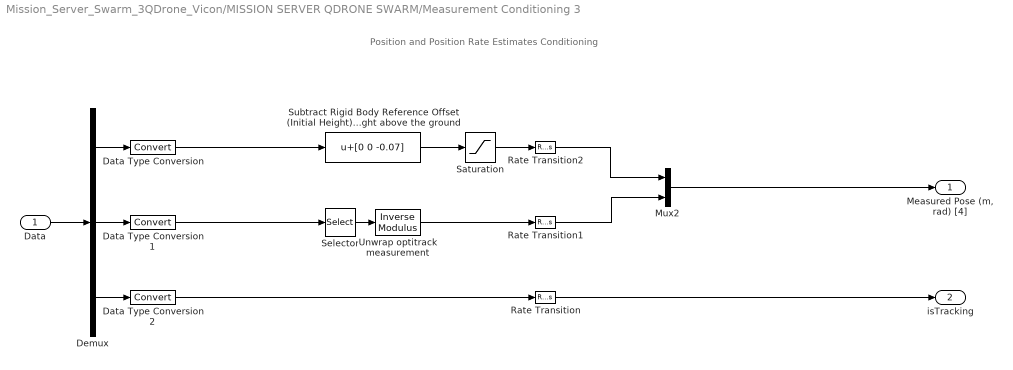
== system Mission_Server_Swarm_3QDrone_Vicon/MISSION SERVER QDRONE SWARM/Measurement Conditioning 3 ==
  note: Position and Position Rate Estimates Conditioning
  Data : Inport
  Data Type Conversion : DataTypeConversion
  Data Type Conversion1 : DataTypeConversion
  Data Type Conversion2 : DataTypeConversion
  Demux : Demux  Outputs=[3 3 1]
  Mux2 : Mux  Inputs=[3 1]
  Rate Transition : RateTransition
  Rate Transition1 : RateTransition
  Rate Transition2 : RateTransition
  Saturation : Saturate  UpperLimit=[2 2 5]  LowerLimit=[-2 -2 0]
  Selector : Selector  InputPortWidth=3  IndexOptions=Index vector (dialog)  Indices=[3]  OutputSizes=1
  Subtract Rigid Body Reference Offset (Initial Height)  to get height above the ground : Bias  Bias=[0 0 -0.07]
  Unwrap optitrack measurement : quarc_library/Discontinuities/Inverse Modulus  modulus=2*pi  output_derivative=off  output_revolutions=off  max_x=Inf  min_x=-Inf
  "Measured Pose (m, rad) [4]" : Outport  VectorParamsAs1DForOutWhenUnconnected=off
  isTracking : Outport  Port=2  VectorParamsAs1DForOutWhenUnconnected=off
  wires:
  Demux/2 -> Data Type Conversion1/1
  Demux/1 -> Data Type Conversion/1
  Demux/3 -> Data Type Conversion2/1
  Mux2/1 -> "Measured Pose (m, rad) [4]"/1
  Data Type Conversion2/1 -> Rate Transition/1
  Data/1 -> Demux/1
  Rate Transition/1 -> isTracking/1
  Subtract Rigid Body Reference Offset (Initial Height)  to get height above the ground/1 -> Saturation/1
  Rate Transition2/1 -> Mux2/1
  Saturation/1 -> Rate Transition2/1
  Data Type Conversion1/1 -> Selector/1
  Selector/1 -> Unwrap optitrack measurement/1
  Data Type Conversion/1 -> Subtract Rigid Body Reference Offset (Initial Height)  to get height above the ground/1
  Unwrap optitrack measurement/1 -> Rate Transition1/1
  Rate Transition1/1 -> Mux2/2

== system Mission_Server_Swarm_3QDrone_Vicon/MISSION SERVER QDRONE SWARM/Subsystem ==
  note: Pass along the communication issue flag only after the connection with the vehicle model was established.
  Communication Issue (0,1) : Inport
  Demux : Demux  Outputs=3
  Logical Operator : Logic  Operator=OR  Inputs=1  AllPortsSameDT=off  OutDataTypeStr=boolean
  Mux : Mux  Inputs=3
  Product : Product
  Product1 : Product
  Product2 : Product
  Show Message on Host : quarc_library/Sinks/Error Handling/Show Message on Host  message_type=Fixed error message  message_icon=Warning  message=Mission Server: Communication Issue with a QDrone
      settings: AttributesFormatString="\"%<message>\""  SourceProductName=QUARC Targets
  Triggered Subsystem : Subsystem  TreatAsAtomicUnit=on
  Triggered Subsystem1 : Subsystem  TreatAsAtomicUnit=on
  Triggered Subsystem2 : Subsystem  TreatAsAtomicUnit=on
  Comm Issue : Outport  VectorParamsAs1DForOutWhenUnconnected=off
  wires:
  Communication Issue (0,1)/1 -> Demux/1
  Demux/1 -> Product/1, Triggered Subsystem/Trigger
  Demux/2 -> Product1/1, Triggered Subsystem1/Trigger
  Demux/3 -> Product2/1, Triggered Subsystem2/Trigger
  Triggered Subsystem/1(Communication Issue (0,1)) -> Product/2
  Triggered Subsystem2/1(Communication Issue (0,1)) -> Product2/2
  Triggered Subsystem1/1(Communication Issue (0,1)) -> Product1/2
  Product2/1 -> Mux/3
  Product1/1 -> Mux/2
  Product/1 -> Mux/1
  Mux/1 -> Logical Operator/1, Comm Issue/1
  Logical Operator/1 -> Show Message on Host/1

== system Mission_Server_Swarm_3QDrone_Vicon/MISSION SERVER QDRONE SWARM/calculate loop back time ==
  Timestamp sent (s) : Inport
  Timestamps received (s) [3] : Inport  Port=2
  Demux : Demux  Outputs=3
  Mux : Mux  Inputs=3
  Subtract : Sum  Inputs=+-
  Subtract1 : Sum  Inputs=+-
  Subtract2 : Sum  Inputs=+-
  Loop Back Tmes (s) [3] : Outport  VectorParamsAs1DForOutWhenUnconnected=off
  wires:
  Timestamp sent (s)/1 -> Subtract1/1, Subtract2/1, Subtract/1
  Timestamps received (s) [3]/1 -> Demux/1
  Demux/1 -> Subtract/2
  Demux/2 -> Subtract1/2
  Demux/3 -> Subtract2/2
  Subtract/1 -> Mux/1
  Subtract1/1 -> Mux/2
  Subtract2/1 -> Mux/3
  Mux/1 -> Loop Back Tmes (s) [3]/1
